simulink model "A00_Basic"  (R2016a)
settings: Solver=VariableStepAuto  StartTime=0.0  StopTime=1500  RelTol=1e-3
libraries: realtime_pacer_lib x1
settings Model: Creator=tiago  LastModifiedBy=tiago

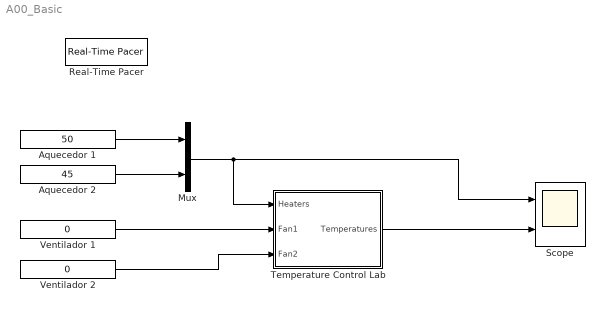
== system A00_Basic ==
  Aquecedor 1 : Constant  Value=50
  Aquecedor 2 : Constant  Value=45
  Mux : Mux  Inputs=2
  Real-Time Pacer : realtime_pacer_lib/Real-Time Pacer  simTimePerRealTime=1
  Scope : Scope  NumInputPorts=2
  Temperature Control Lab : Subsystem
      mask Display: image('tclab.png');
  Ventilador 1 : Constant  Value=0
  Ventilador 2 : Constant  Value=0
  wires:
  Ventilador 1/1 -> Temperature Control Lab/2(Fan1)
  Ventilador 2/1 -> Temperature Control Lab/3(Fan2)
  Mux/1 -> Scope/1, Temperature Control Lab/1(Heaters)
  Aquecedor 1/1 -> Mux/1
  Aquecedor 2/1 -> Mux/2
  Temperature Control Lab/1(Temperatures) -> Scope/2

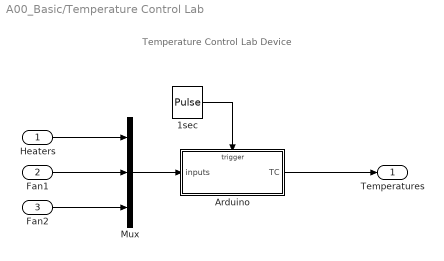
== system A00_Basic/Temperature Control Lab ==
  note: Temperature Control Lab Device
  Heaters : Inport  PortDimensions=2
  Fan1 : Inport  Port=2  PortDimensions=1
  Fan2 : Inport  Port=3  PortDimensions=1
  1sec : DiscretePulseGenerator  PulseType=Time based  Period=0.5  PulseWidth=50
  Arduino : Subsystem  TreatAsAtomicUnit=on
  Mux : Mux  Inputs=3
  Temperatures : Outport
  wires:
  1sec/1 -> Arduino/Trigger
  Arduino/1(TC) -> Temperatures/1
  Mux/1 -> Arduino/1(inputs)
  Heaters/1 -> Mux/1
  Fan2/1 -> Mux/3
  Fan1/1 -> Mux/2

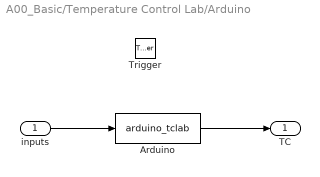
== system A00_Basic/Temperature Control Lab/Arduino ==
  inputs : Inport  PortDimensions=4  LatchByDelayingOutsideSignal=on
  Trigger : TriggerPort  VariantControl=Variant
  Arduino : MATLABFcn  MATLABFcn=arduino_tclab
  TC : Outport  InitialOutput=[23 23]
  wires:
  inputs/1 -> Arduino/1
  Arduino/1 -> TC/1
